simulink library "libwind"  (R2022a)
settings: Solver=ode45  StartTime=0.0  StopTime=10.0  RelTol=1e-3  EnableMultiTasking=on
settings Model: Creator=grunnet  LastModifiedBy=yerai
settings SolverCC: AlgebraicLoopSolver=TrustRegion
settings DataIOCC: LimitDataPoints=on  SaveFormat=Array  SignalLoggingSaveFormat=ModelDataLogs  ReturnWorkspaceOutputs=off
settings OptimizationCC: ExpressionDepthLimit=2147483647  LifeSpan=inf
settings DebuggingCC: UnderspecifiedInitializationDetection=Classic  MergeDetectMultiDrivingBlocksExec=none  SolverPrmCheckMsg=warning  FcnCallInpInsideContextMsg=warning  UnconnectedInputMsg=warning  UnconnectedOutputMsg=warning  UnconnectedLineMsg=warning  StateNameClashWarn=warning  SFUnexpectedBacktrackingDiag=warning  SFNoUnconditionalDefaultTransitionDiag=warning  SFExecutionAtInitializationDiag=none  SFMachineParentedDataDiag=warning  ArithmeticOperatorsInVariantConditions=warning
settings HardwareCC: ProdBitPerPointer=32  ProdBitPerSizeT=32  ProdBitPerPtrDiffT=32  ProdLargestAtomicFloat=None  ProdIntDivRoundTo=Undefined  ProdEndianess=Unspecified  ProdWordSize=32  ProdHWDeviceType=32-bit Generic
settings ModelReferenceCC: PropagateSignalLabelsOutOfModel=off
settings SFSimCC: SimUseLocalCustomCode=off  CustomCodeUndefinedFunction=UseInterfaceOnly
settings RTWCC: RTWUseLocalCustomCode=off  DLArmComputeVersion=19.05
settings CodeAppCC: StateflowObjectComments=on
settings GRTTargetCC: TargetLangStandard=C89/C90 (ANSI)  CombineOutputUpdateFcns=off  GRTInterface=on
settings ConfigComp: CovMetricSettings=dw  CovSaveCumulativeToWorkspaceVar=on  CovSaveSingleToWorkspaceVar=on  CovExternalEMLEnable=off

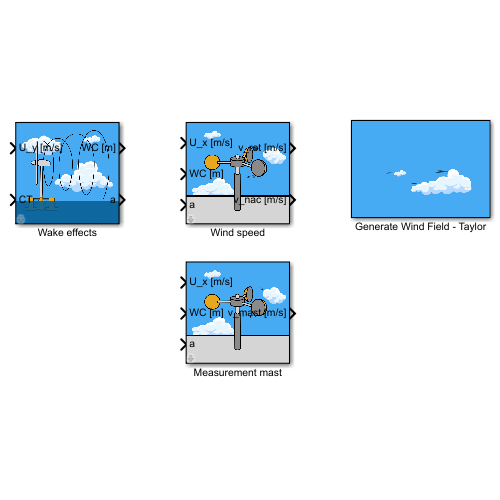
[thumbnail: Simulink's stored preview of the top-level diagram]
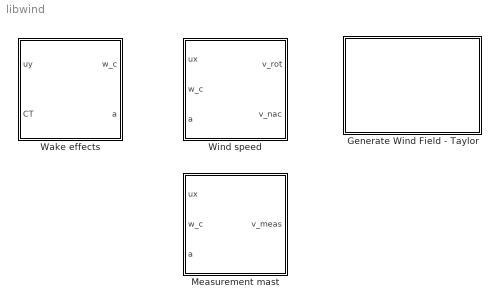
== system libwind ==
  Generate Wind Field - Taylor : Subsystem  mask(Wind field generation){}
      mask help: Generates a wind field
      settings: OpenFcn=create_windfield()
      mask Display: image(imread('wind.png'))
  Measurement mast : Subsystem  AncestorBlock=libwind/Wind speed  mask(Wind){}
      mask help: Calculates average over rotor and nacelle wind speeds based on wake effects
      mask init:
      | p=get_param(gcb,'UserData');
      mask Display:
      | image(imread('wind_speed.png'))
      | 
      | port_label('output',1,'v_mast [m/s]')
      | 
      | port_label('input',1,'U_x [m/s]')
      | port_label('input',2,'WC [m]')
      | port_label('input',3,'a')
  Wake effects : Subsystem  mask(Wind){}
      mask help: Calculates wake effects based on turbine CT and crosswinds
      mask init:
      | p=get_param(gcb,'UserData');
      mask Display:
      | image(imread('wind_wake.png'))
      | 
      | port_label('output',1,'WC [m]')
      | port_label('output',2,'a')
      | 
      | 
      | port_label('input',1,'U_y [m/s]')
      | port_label('input',2,'CT')
  Wind speed : Subsystem  mask(Wind){}
      mask help: Calculates average over rotor and nacelle wind speeds based on wake effects
      mask init:
      | p=get_param(gcb,'UserData');
      mask Display:
      | image(imread('wind_speed.png'))
      | 
      | port_label('output',1,'v_rot [m/s]')
      | port_label('output',2,'v_nac [m/s]')
      | 
      | 
      | port_label('input',1,'U_x [m/s]')
      | port_label('input',2,'WC [m]')
      | port_label('input',3,'a')

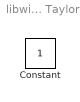
== system libwind/Generate Wind Field - Taylor ==
  Constant : Constant

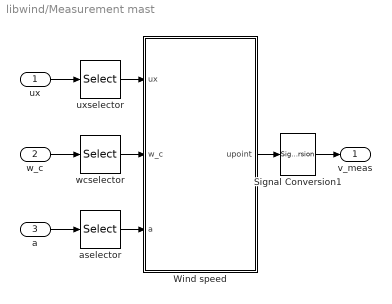
== system libwind/Measurement mast ==
  ux : Inport
  w_c : Inport  Port=2
  a : Inport  Port=3
  Signal Conversion1 : SignalConversion  ConversionOutput=Contiguous copy  OverrideOpt=off
  Wind speed : MATLAB Function  TreatAsAtomicUnit=on
  aselector : Selector  NumberOfDimensions=2  InputPortWidth=3  IndexOptions=Index vector (dialog),Select all  Indices=p.mast.num,p.wt.num  OutputSizes=1,1
  uxselector : Selector  NumberOfDimensions=2  InputPortWidth=3  IndexOptions=Select all,Index vector (dialog)  Indices=[1 3],p.mast.num  OutputSizes=1,1
  wcselector : Selector  NumberOfDimensions=2  InputPortWidth=3  IndexOptions=Index vector (dialog),Select all  Indices=p.mast.num,p.wt.num  OutputSizes=1,1
  v_meas : Outport
  wires:
  Signal Conversion1/1 -> v_meas/1
  uxselector/1 -> Wind speed/1(ux)
  aselector/1 -> Wind speed/3(a)
  a/1 -> aselector/1
  wcselector/1 -> Wind speed/2(w_c)
  w_c/1 -> wcselector/1
  ux/1 -> uxselector/1
  Wind speed/1(upoint) -> Signal Conversion1/1

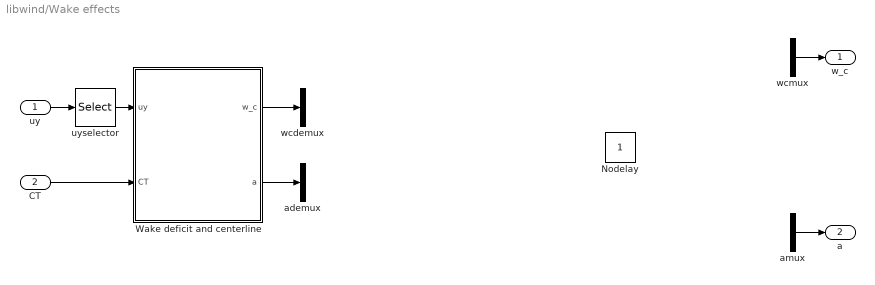
== system libwind/Wake effects ==
  uy : Inport
  CT : Inport  Port=2
  Nodelay : Constant
  Wake deficit and centerline : MATLAB Function  TreatAsAtomicUnit=on
  ademux : Demux  Outputs=2
  amux : Mux  Inputs=2
  uyselector : Selector  NumberOfDimensions=2  InputPortWidth=3  IndexOptions=Select all,Index vector (dialog)  Indices=[1 3],p.wt.num  OutputSizes=1,1
  wcdemux : Demux  Outputs=2
  wcmux : Mux  Inputs=2
  w_c : Outport
  a : Outport  Port=2
  wires:
  CT/1 -> Wake deficit and centerline/2(CT)
  uy/1 -> uyselector/1
  uyselector/1 -> Wake deficit and centerline/1(uy)
  Wake deficit and centerline/1(w_c) -> wcdemux/1
  Wake deficit and centerline/2(a) -> ademux/1
  wcmux/1 -> w_c/1
  amux/1 -> a/1

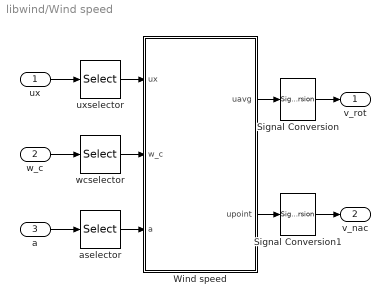
== system libwind/Wind speed ==
  ux : Inport
  w_c : Inport  Port=2
  a : Inport  Port=3
  Signal Conversion : SignalConversion  ConversionOutput=Contiguous copy  OverrideOpt=off
  Signal Conversion1 : SignalConversion  ConversionOutput=Contiguous copy  OverrideOpt=off
  Wind speed : MATLAB Function  TreatAsAtomicUnit=on
  aselector : Selector  NumberOfDimensions=2  InputPortWidth=3  IndexOptions=Index vector (dialog),Select all  Indices=p.wt.num,p.wt.num  OutputSizes=1,1
  uxselector : Selector  NumberOfDimensions=2  InputPortWidth=3  IndexOptions=Select all,Index vector (dialog)  Indices=[1 3],p.wt.num  OutputSizes=1,1
  wcselector : Selector  NumberOfDimensions=2  InputPortWidth=3  IndexOptions=Index vector (dialog),Select all  Indices=p.wt.num,p.wt.num  OutputSizes=1,1
  v_rot : Outport
  v_nac : Outport  Port=2
  wires:
  Wind speed/2(upoint) -> Signal Conversion1/1
  Wind speed/1(uavg) -> Signal Conversion/1
  ux/1 -> uxselector/1
  w_c/1 -> wcselector/1
  wcselector/1 -> Wind speed/2(w_c)
  a/1 -> aselector/1
  aselector/1 -> Wind speed/3(a)
  uxselector/1 -> Wind speed/1(ux)
  Signal Conversion/1 -> v_rot/1
  Signal Conversion1/1 -> v_nac/1

== matlab function libwind/Measurement mast/Wind speed ==
  data: ux input; w_c input; a input; p parameter; upoint output
function upoint  = windspeed(ux,w_c,a,p)
%     ux    is the wind vector at the x position of the turbine
%     w_c   is the vector of wake centers from the other turbins at the x position of the turbine
%     a     is the vector of velocity deficits at this turbine from the other turbines
%     P     is a structure containing parameters  
       
% %     Initialise variables
    av = ones(p.grid.ysize,1);
% %     Merge the wake from all turbines upwind
    for i = 1:length(p.farm.x)
        if(p.farm.x(i) < p.mast.x) % Only compute deficit effect from upstream turbines
% %             Compute the grid number for low meandering edge
            mn              = floor((w_c(i)-p.wt.exprad(i))/p.grid.size)+1;
            m_min           = max(mn,1); 
% %             Compute the grid number for the high meandering edge
            mx              = floor((w_c(i)+p.wt.exprad(i))/p.grid.size)+1;
            m_max           = min(mx,floor(p.grid.ysize/p.grid.size)+1);
% %             Merge wakes
            for j = m_min:m_max
                av(j) = av(j)*a(i);
            end
        end
    end
    
% %     Extract the wake corrected velocity at the nacelle
    upoint  = ux(floor(p.mast.y/p.grid.size)+1)*av(floor(p.mast.y/p.grid.size)+1);
end

== matlab function libwind/Wake effects/Wake deficit and centerline ==
  data: uy input; CT input; p parameter; w_c output; a output
function [w_c,a] = wake(uy,CT,p)
% %     Todo: Change length(uy)*grid_size to farm size?
% %           Change such that parm is passed directly

    w_c = zeros(length(p.farm.xTot),1);
    a   = ones(length(p.farm.xTot),1);
    
% %     Find wake center and deficit for all other turbines/masts
    for i = 1:length(p.farm.xTot)
        if(p.farm.xTot(i)-p.wt.x > 0)  % Only if when the turbine/mast is downwind
            w_c(i)  = max(min(wakecenter(uy,p.farm.xTot(i),p),p.grid.ysize),1);
            a(i)    = deficit(CT,p.farm.xTot(i),p);
        else
            w_c(i)  = p.wt.y;
            a(i)    = 1;
        end
    end
end


function wc = wakecenter(uy,px,p)
    it = ceil((px-p.wt.x)/p.grid.size);     % Compute number of grid points to px
    wc = p.wt.y;                            % Wake center starts at turbine position
    
    for i = 1:it % Compute the meandering for each grid point
% %         Compute the grid number for low meandering edge
        m_min = max(floor((wc-p.wt.meand.r(i))/p.grid.size)+1,1); 
% %         Compute the grid number for the high meandering edge
        m_max = min(ceil((wc+p.wt.meand.r(i))/p.grid.size)+1,length(uy)); 
        
% %         Average transversal velocity over the wake area
        uysum = 0;
        for j = m_min:m_max
            uysum = uysum+uy(j);
        end
        uyavg = uysum/(m_max-m_min+1);
        
% %         Notice here ts such that wake moves with uyavg speed
        wc    = wc+p.ts*uyavg;
    end
end

function a = deficit(CT,px,p) % Wake deficit at px-wtx distance from turbine
    a = 1-.5*CT/(1+(px-p.wt.x)/(4*p.wt.rotor.r));
end

== matlab function libwind/Wind speed/Wind speed ==
  data: uavg output; ux input; w_c input; a input; p parameter; upoint output
function [uavg,upoint] = windspeed(ux,w_c,a,p)
%     ux    is the wind vector at the x position of the turbine
%     w_c   is the vector of wake centers from the other turbins at the x position of the turbine
%     a     is the vector of velocity deficits at this turbine from the other turbines
%     P     is a structure containing parameters  
       
% %     Initialise variables
    av = ones(p.grid.ysize,1);
% %     Merge the wake from all turbines upwind
    for i = 1:length(p.farm.x)
        if(p.farm.x(i) < p.wt.x) % Only compute deficit effect from upstream turbines
% %             Compute the grid number for low meandering edge
            mn              = floor((w_c(i)-p.wt.exprad(i))/p.grid.size)+1;
            m_min           = max(mn,1); 
% %             Compute the grid number for the high meandering edge
            mx              = floor((w_c(i)+p.wt.exprad(i))/p.grid.size)+1;
            m_max           = min(mx,floor(p.grid.ysize/p.grid.size)+1);
% %             Merge wakes
            for j = m_min:m_max
                av(j) = av(j)*a(i);
            end
        end
    end
    
% %     Rotor grid points - Todo move to farm setup
% %     compute the grid number for low rotor edge
    r_min   = floor((p.wt.y-p.wt.rotor.r)/p.grid.size)+1; 
% %     compute the grid number for the high rotor edge
    r_max   = floor((p.wt.y+p.wt.rotor.r)/p.grid.size)+1;
    
% %     Compute the average of the wake corrected x-velocities over the rotor dish area
    uavg   = mean(ux(r_min:r_max).*av(r_min:r_max));
    
% %     Extract the wake corrected velocity at the nacelle
    upoint  = ux(floor(p.wt.y/p.grid.size)+1)*av(floor(p.wt.y/p.grid.size)+1);
end
